simulink model "motor"  (R2025a)
settings: Solver=VariableStepAuto  StartTime=0.0  StopTime=10.0  RelTol=1e-3
values from neighbouring files (symbols this model uses):
  CM_FRIC = [ ... (first row only)    [motor parameter.m]
  J = 9e-7    (= 9e-07)    [motor parameter.m]
  L_A = 0.015    [motor parameter.m]
  R_A = 8    [motor parameter.m]
undefined symbols (not defined in the file or in its folder): k_G
settings Model: Creator=kavin  LastModifiedBy=kavin

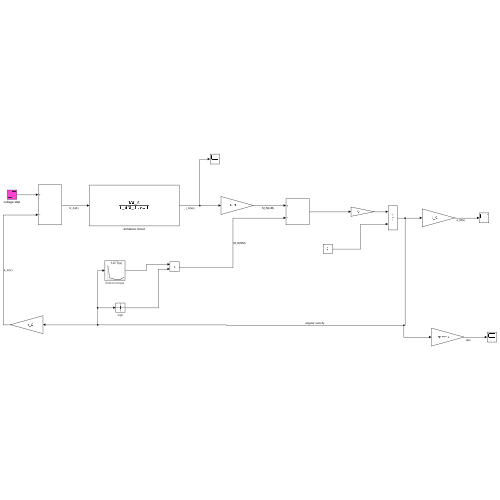
[thumbnail: Simulink's stored preview of the top-level diagram]
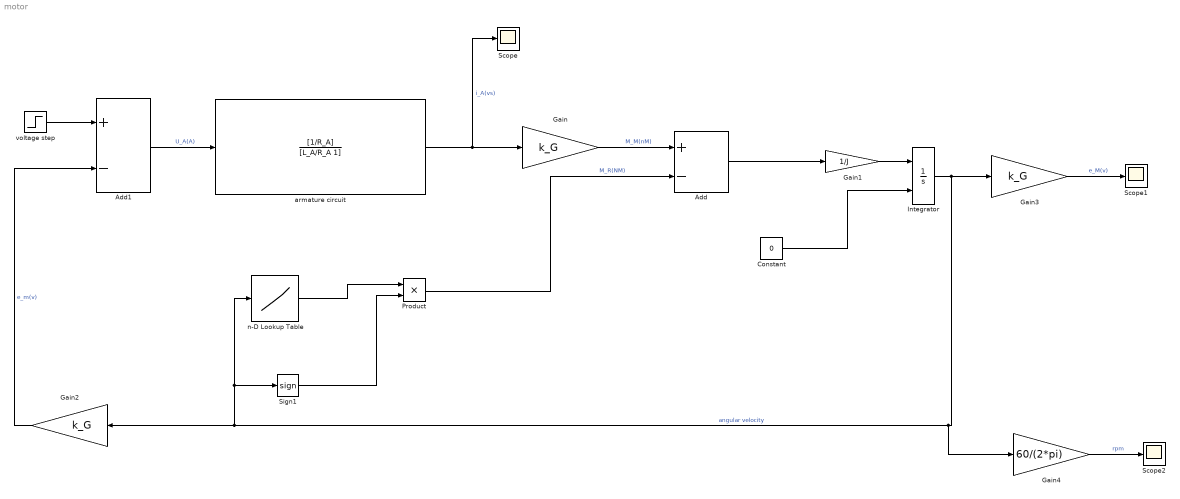
== system motor ==
  Add : Sum  Inputs=+-
  Add1 : Sum  Inputs=+-
  Constant : Constant  Value=0
  Gain : Gain  Gain=k_G
  Gain1 : Gain  Gain=1/J
  Gain2 : Gain  Gain=k_G
  Gain3 : Gain  Gain=k_G
  Gain4 : Gain  Gain=60/(2*pi)
  Integrator : Integrator  InitialConditionSource=external
  Product : Product
  Scope : Scope
      settings: ActiveDisplayYMinimum=-1  ActiveDisplayYMaximum=1
  Scope1 : Scope
      settings: ActiveDisplayYMinimum=-1  ActiveDisplayYMaximum=1
  Scope2 : Scope
      settings: ActiveDisplayYMinimum=-1  ActiveDisplayYMaximum=1  DataLoggingVariableName=ScopeData2
  Sign1 : Signum
      settings: AttributesFormatString=sign
  armature circuit : TransferFcn  Numerator=[1/R_A]  Denominator=[L_A/R_A 1]
  n-D Lookup Table : Lookup_n-D  NumberOfTableDimensions=1  BreakpointsForDimension1=CM_FRIC(1,:)  BreakpointsForDimension3=[5, 7]  Table=CM_FRIC(2,:)  InternalRulePriority=Speed  RndMeth=Simplest
      settings: AttributesFormatString=friction torque
  voltage step : Step  After=5  SampleTime=0
  wires:
  voltage step/1 -> Add1/1
  Gain/1 -> Add/1  "M_M(nM)"
  armature circuit/1 -> Scope/1, Gain/1  "i_A(vs)"
  Add1/1 -> armature circuit/1  "U_A(A)"
  Product/1 -> Add/2  "M_R(NM)"
  n-D Lookup Table/1 -> Product/1
  Sign1/1 -> Product/2
  Add/1 -> Gain1/1
  Gain1/1 -> Integrator/1
  Constant/1 -> Integrator/2
  Gain2/1 -> Add1/2  "e_m(v)"
  Integrator/1 -> Gain4/1, Sign1/1, n-D Lookup Table/1, Gain2/1, Gain3/1  "angular velocity"
  Gain3/1 -> Scope1/1  "e_M(v)"
  Gain4/1 -> Scope2/1  "rpm"
